simulink subsystem "COMP_QUAD_COL_SYS_B"  (R2025b)
settings: Solver=VariableStepAuto  StartTime=0.0  StopTime=10.0  RelTol=1e-3
undefined symbols (not defined in the file): X, Y, Z
libraries: sm_lib x16
settings Model: Creator=bhorton  LastModifiedBy=bhorton

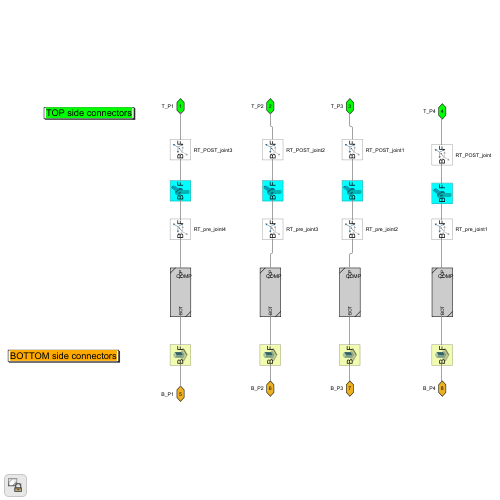
[thumbnail: Simulink's stored preview of the top-level diagram]
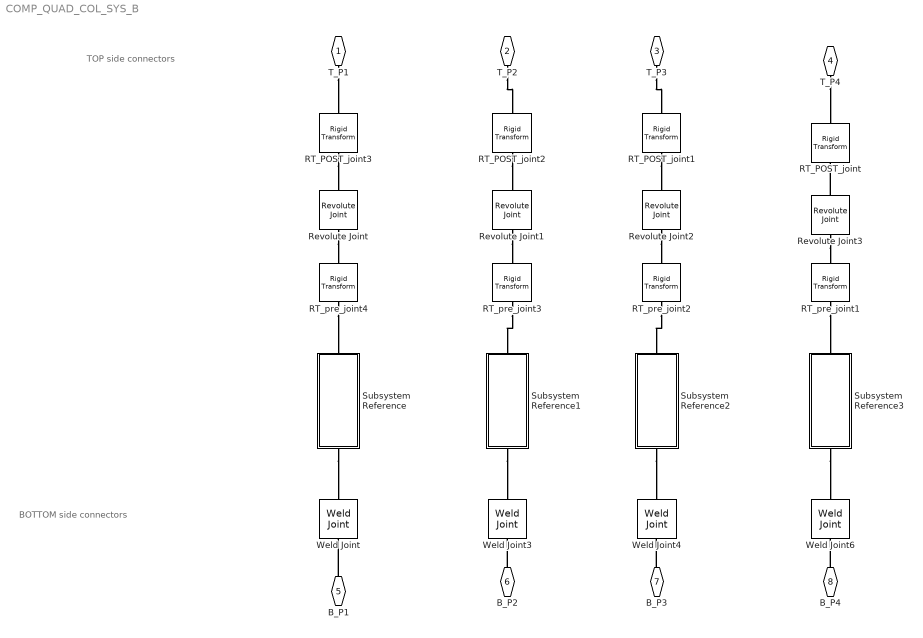
== system COMP_QUAD_COL_SYS_B ==
  note: TOP side connectors
  note: BOTTOM side connectors
  RT_POST_joint{,1..3} (4 alike) : sm_lib/Frames and Transforms/Rigid Transform  RotationMethod=AlignedAxes  FollAlignAxisA=+X  BaseAlignAxisA=+X  FollAlignAxisB=+Z  BaseAlignAxisB=+Y  RotationStandardAxis=+Z  RotationAngle=0  RotationAngleUnits=deg  RotationArbitraryAxis=[0 0 1]  RotationSequenceAxes=FollowerAxes  RotationSequence=XYX  RotationSequenceAngles=[0 0 0]  RotationSequenceAnglesUnits=deg  RotationMatrix=[1 0 0;0 1 0;0 0 1]  Quaternion=[1 0 0 0]  TranslationMethod=None  TranslationCartesianOffset=[0 0 0]  TranslationCartesianOffsetUnits=m  TranslationStandardAxis=+Z  TranslationStandardOffset=0  TranslationStandardOffsetUnits=m  TranslationROffset=0  TranslationROffsetUnits=m  TranslationThetaOffset=0  TranslationThetaOffsetUnits=deg  TranslationZOffset=0  TranslationZOffsetUnits=m
  RT_pre_joint{1..4} (4 alike) : sm_lib/Frames and Transforms/Rigid Transform  RotationMethod=AlignedAxes  FollAlignAxisA=+X  BaseAlignAxisA=+X  FollAlignAxisB=+Y  BaseAlignAxisB=+Z  RotationStandardAxis=+Z  RotationAngle=0  RotationAngleUnits=deg  RotationArbitraryAxis=[0 0 1]  RotationSequenceAxes=FollowerAxes  RotationSequence=XYX  RotationSequenceAngles=[0 0 0]  RotationSequenceAnglesUnits=deg  RotationMatrix=[1 0 0;0 1 0;0 0 1]  Quaternion=[1 0 0 0]  TranslationMethod=None  TranslationCartesianOffset=[0 0 0]  TranslationCartesianOffsetUnits=m  TranslationStandardAxis=+Z  TranslationStandardOffset=0  TranslationStandardOffsetUnits=m  TranslationROffset=0  TranslationROffsetUnits=m  TranslationThetaOffset=0  TranslationThetaOffsetUnits=deg  TranslationZOffset=0  TranslationZOffsetUnits=m
  Revolute Joint{,1..3} (4 alike) : sm_lib/Joints/Revolute Joint  JointMode=Normal  CompositeWrenchDir=FollowerOnBase  CompositeWrenchFrame=BaseFrame  SenseConstraintForce=off  SenseConstraintTorque=off  SenseTotalForce=off  SenseTotalTorque=off  PositionTargetSpecify=off  PositionTargetPriority=High  PositionTargetValue=0  PositionTargetValueUnits=deg  VelocityTargetSpecify=off  VelocityTargetPriority=High  VelocityTargetValue=0  VelocityTargetValueUnits=deg/s  EquilibriumPosition=0  EquilibriumPositionUnits=deg  SpringStiffness=0  SpringStiffnessUnits=N*m/deg  DampingCoefficient=0  DampingCoefficientUnits=N*m/(deg/s)  LowerLimitSpecify=off  LowerLimitBound=-90  LowerLimitBoundUnits=deg  LowerLimitStiffness=1e4  LowerLimitStiffnessUnits=N*m/deg  LowerLimitDamping=10  LowerLimitDampingUnits=N*m/(deg/s)  LowerLimitTransitionRegionWidth=0.1  LowerLimitTransitionRegionWidthUnits=deg  UpperLimitSpecify=off  UpperLimitBound=90  UpperLimitBoundUnits=deg  UpperLimitStiffness=1e4  UpperLimitStiffnessUnits=N*m/deg  UpperLimitDamping=10  UpperLimitDampingUnits=N*m/(deg/s)  UpperLimitTransitionRegionWidth=0.1  UpperLimitTransitionRegionWidthUnits=deg  TorqueActuationMode=NoTorque  MotionActuationMode=ComputedMotion  SensePosition=off  SenseVelocity=off  SenseAcceleration=off  SenseTorqueForce=off  SenseLowerLimitTorqueForce=off  SenseUpperLimitTorqueForce=off
  Subsystem Reference{,1..3} (4 alike) : Subsystem  ReferencedSubsystem=COMP_COL_SYS
  Weld Joint{,3..4,6} (4 alike) : sm_lib/Joints/Weld Joint  JointMode=Normal  CompositeWrenchDir=FollowerOnBase  CompositeWrenchFrame=BaseFrame  SenseConstraintForce=off  SenseConstraintTorque=off  SenseTotalForce=off  SenseTotalTorque=off
  T_P1 : PMIOPort  Side=Left
  T_P2 : PMIOPort  Port=2  Side=Left
  T_P3 : PMIOPort  Port=3  Side=Left
  T_P4 : PMIOPort  Port=4  Side=Left
  B_P1 : PMIOPort  Port=5  Side=Right
  B_P2 : PMIOPort  Port=6  Side=Right
  B_P3 : PMIOPort  Port=7  Side=Right
  B_P4 : PMIOPort  Port=8  Side=Right
  connections:
  Subsystem Reference/RConn1 -- Weld Joint/RConn1
  B_P4/RConn1 -- Weld Joint6/LConn1
  B_P3/RConn1 -- Weld Joint4/LConn1
  Subsystem Reference3/RConn1 -- Weld Joint6/RConn1
  Subsystem Reference2/RConn1 -- Weld Joint4/RConn1
  Subsystem Reference1/RConn1 -- Weld Joint3/RConn1
  B_P1/RConn1 -- Weld Joint/LConn1
  B_P2/RConn1 -- Weld Joint3/LConn1
  RT_pre_joint4/LConn1 -- Subsystem Reference/LConn1
  RT_pre_joint3/LConn1 -- Subsystem Reference1/LConn1
  RT_pre_joint2/LConn1 -- Subsystem Reference2/LConn1
  RT_pre_joint1/LConn1 -- Subsystem Reference3/LConn1
  Revolute Joint1/LConn1 -- RT_pre_joint3/RConn1
  Revolute Joint/LConn1 -- RT_pre_joint4/RConn1
  Revolute Joint2/LConn1 -- RT_pre_joint2/RConn1
  Revolute Joint3/LConn1 -- RT_pre_joint1/RConn1
  Revolute Joint3/RConn1 -- RT_POST_joint/LConn1
  RT_POST_joint1/LConn1 -- Revolute Joint2/RConn1
  RT_POST_joint2/LConn1 -- Revolute Joint1/RConn1
  RT_POST_joint3/LConn1 -- Revolute Joint/RConn1
  T_P4/RConn1 -- RT_POST_joint/RConn1
  T_P3/RConn1 -- RT_POST_joint1/RConn1
  T_P2/RConn1 -- RT_POST_joint2/RConn1
  T_P1/RConn1 -- RT_POST_joint3/RConn1
